simulink model "digital_subsystem_wrapper"  (R2024a)
settings: Solver=VariableStepAuto  StartTime=0.0  StopTime=1  MaxStep=Ts/10
PreLoadFcn:
  | s0=sprintf('===========================================================================');disp(s0)
  | s1=sprintf('= Created by Bader Almutair bmutairi@kacst.edu.sa                         =');disp(s1)
  | s2=sprintf('= Date 12/11/2014                                                         =');disp(s2)
  | s3=sprintf('= Refer to the PhD thesis Ch4,P.55                                        =');disp(s3)
  | s4=sprintf('===========================================================================');disp(s4)
values from neighbouring files (symbols this model uses):
  inject_signal_enable = 0    [simon_test.m]    (also in testPSD_simulink.m)
  Ts = 1/Fs    (= 7.50007500075e-06)    [new_generation_coeff.m]    (also in simon_test.m; simple_fft_test.m = 1/F; testPSD_c2d.m; testPSD_simulink.m)
undefined symbols (not defined in the file or in its folder): D2den, D2num, Digital_Compv2_den, Digital_Compv2_num
settings Model: DataTypeOverride=Off  Creator=Administrator  LastModifiedBy=Simon
settings SolverCC: AlgebraicLoopSolver=TrustRegion
settings DataIOCC: LimitDataPoints=on  SaveFormat=Array  SaveOutput=off  SaveTime=off  ReturnWorkspaceOutputs=off
settings OptimizationCC: BlockReduction=off  ConditionallyExecuteInputs=off  DefaultParameterBehavior=Inlined  InheritOutputTypeSmallerThanSingle=on  ReuseModelBlockBuffer=off  ExpressionDepthLimit=2147483647  LifeSpan=inf
settings DebuggingCC: AlgebraicLoopMsg=error  UnderspecifiedInitializationDetection=Classic  MergeDetectMultiDrivingBlocksExec=none  SolverPrmCheckMsg=warning  SingleTaskRateTransMsg=error  FcnCallInpInsideContextMsg=warning  UnconnectedInputMsg=warning  UnconnectedOutputMsg=warning  UnconnectedLineMsg=warning  StateNameClashWarn=warning  SFUnexpectedBacktrackingDiag=warning  SFNoUnconditionalDefaultTransitionDiag=warning  SFExecutionAtInitializationDiag=none  ArithmeticOperatorsInVariantConditions=warning
settings HardwareCC: ProdBitPerPointer=32  ProdBitPerSizeT=32  ProdBitPerPtrDiffT=32  ProdLargestAtomicFloat=None  ProdIntDivRoundTo=Undefined  ProdEndianess=Unspecified  ProdWordSize=32  ProdHWDeviceType=ASIC/FPGA->ASIC/FPGA  TargetBitPerPointer=64  TargetBitPerSizeT=64  TargetBitPerPtrDiffT=64  TargetLongLongMode=on  TargetIntDivRoundTo=Zero  TargetEndianess=LittleEndian  TargetWordSize=64  TargetHWDeviceType=Custom Processor->MATLAB Host Computer  ProdEqTarget=off
settings ModelReferenceCC: PropagateSignalLabelsOutOfModel=off
settings SFSimCC: SimUseLocalCustomCode=off  CustomCodeUndefinedFunction=UseInterfaceOnly
settings RTWCC: RTWUseLocalCustomCode=off  GPUComputeCapability=3.5
settings CodeAppCC: StateflowObjectComments=on
settings GRTTargetCC: TargetLangStandard=C89/C90 (ANSI)  CombineOutputUpdateFcns=off  GRTInterface=on
settings ConfigComp: CovMetricSettings=dw  CovSaveCumulativeToWorkspaceVar=on  CovSaveSingleToWorkspaceVar=on  CovExternalEMLEnable=off

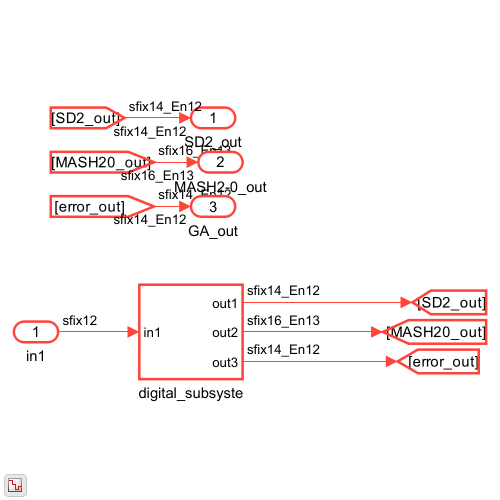
[thumbnail: Simulink's stored preview of the top-level diagram]
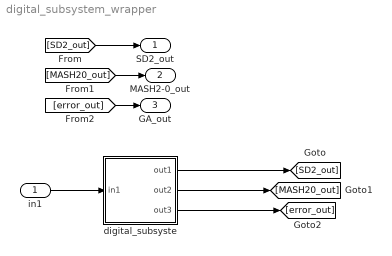
== system digital_subsystem_wrapper ==
  in1 : Inport  OutDataTypeStr=fixdt(1,12,0)  PortDimensions=1  SampleTime=[7.5000750007500074e-06,0]
  digital_subsyste : Subsystem
  SD2_out : Outport  PortDimensions=1  SampleTime=[7.5000750007500074e-06,0]
  MASH2-0_out : Outport  Port=2  PortDimensions=1  SampleTime=[7.5000750007500074e-06,0]
  GA_out : Outport  Port=3  PortDimensions=1  SampleTime=[7.5000750007500074e-06,0]
  wires:
  in1/1 -> digital_subsyste/1(in1)
  digital_subsyste/1(out1) -> [SD2_out]
  digital_subsyste/2(out2) -> [MASH20_out]
  digital_subsyste/3(out3) -> [error_out]
  [SD2_out] -> SD2_out/1
  [MASH20_out] -> MASH2-0_out/1
  [error_out] -> GA_out/1

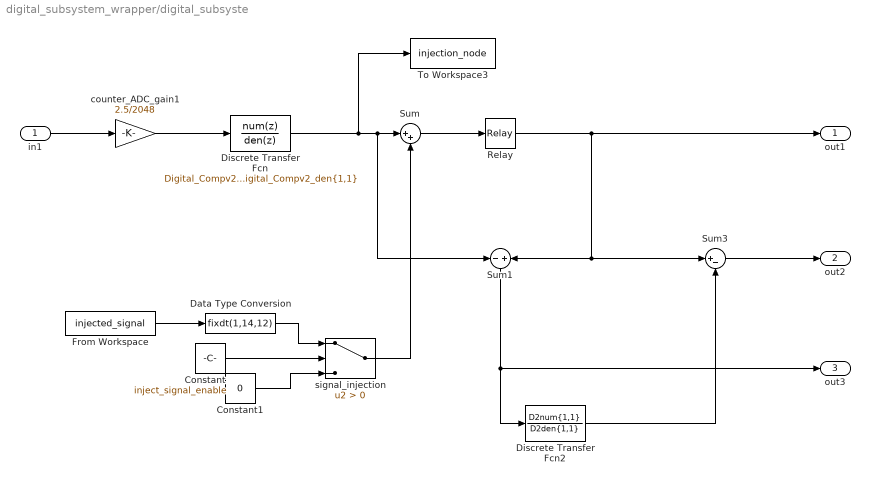
== system digital_subsystem_wrapper/digital_subsyste ==
  in1 : Inport
  Constant : Constant  Value=inject_signal_enable  OutDataTypeStr=boolean  SampleTime=Ts
  Constant1 : Constant  Value=0  OutDataTypeStr=fixdt(1,14,12)  SampleTime=Ts
  Data Type Conversion : DataTypeConversion  OutDataTypeStr=fixdt(1,14,12)  SaturateOnIntegerOverflow=off  RndMeth=Floor
  Discrete Transfer Fcn : DiscreteTransferFcn  Numerator=Digital_Compv2_num{1,1}  Denominator=Digital_Compv2_den{1,1}  NumCoefDataTypeStr=fixdt(1, 64, 32)  DenCoefDataTypeStr=fixdt(1, 64, 32)  NumProductDataTypeStr=fixdt(1, 64, 32)  DenProductDataTypeStr=fixdt(1, 64, 32)  NumAccumDataTypeStr=fixdt(1, 64, 32)  DenAccumDataTypeStr=fixdt(1, 64, 32)  OutDataTypeStr=fixdt(1, 14, 12)  SaturateOnIntegerOverflow=on
  Discrete Transfer Fcn2 : DiscreteTransferFcn  Numerator=D2num{1,1}  Denominator=D2den{1,1}  StateDataTypeStr=fixdt(1, 64, 32)  NumCoefDataTypeStr=fixdt(1, 64, 32)  DenCoefDataTypeStr=fixdt(1, 64, 32)  NumProductDataTypeStr=fixdt(1, 64, 32)  DenProductDataTypeStr=fixdt(1, 64, 32)  NumAccumDataTypeStr=fixdt(1, 64, 32)  DenAccumDataTypeStr=fixdt(1, 64, 32)  OutDataTypeStr=fixdt(1, 18, 15)  SaturateOnIntegerOverflow=on
  From Workspace : FromWorkspace  VariableName=injected_signal  SampleTime=Ts  Interpolate=off  OutputAfterFinalValue=Setting to zero
  Relay : Relay  OnSwitchValue=2^-12  OffSwitchValue=-2^-12  OffOutputValue=-1  OutDataTypeStr=fixdt(1, 14, 12)
  Sum : Sum  Inputs=|++  SaturateOnIntegerOverflow=on  OutDataTypeStr=Inherit: Same as first input
  Sum1 : Sum  Inputs=-+  AccumDataTypeStr=fixdt(1, 64, 32)  InputSameDT=on  OutDataTypeStr=Inherit: Same as first input
  Sum3 : Sum  Inputs=|+-  OutDataTypeStr=fixdt(1, 16, 13)  SaturateOnIntegerOverflow=on
  To Workspace3 : ToWorkspace  VariableName=injection_node  SampleTime=Ts
  counter_ADC_gain1 : Gain  Gain=2.5/2048  OutDataTypeStr=fixdt(1, 14, 12)  SaturateOnIntegerOverflow=on
  signal_injection : Switch  Criteria=u2 > Threshold  SaturateOnIntegerOverflow=off  InputSameDT=off  OutDataTypeStr=Inherit: Same as first input
  out1 : Outport
  out2 : Outport  Port=2
  out3 : Outport  Port=3
  wires:
  Sum3/1 -> out2/1
  Relay/1 -> out1/1, Sum3/1, Sum1/2
  Sum1/1 -> Discrete Transfer Fcn2/1, out3/1
  Discrete Transfer Fcn/1 -> Sum/1, Sum1/1, To Workspace3/1
  in1/1 -> counter_ADC_gain1/1
  counter_ADC_gain1/1 -> Discrete Transfer Fcn/1
  Discrete Transfer Fcn2/1 -> Sum3/2
  Sum/1 -> Relay/1
  signal_injection/1 -> Sum/2
  Constant/1 -> signal_injection/2
  Constant1/1 -> signal_injection/3
  From Workspace/1 -> Data Type Conversion/1
  Data Type Conversion/1 -> signal_injection/1
